simulink model "Simulink"  (R2023b)
settings: Solver=VariableStepAuto  StartTime=0.0  StopTime=1  RelTol=1e-3
undefined symbols (not defined in the file): gray, Rec, SDTV
libraries: visiongeotforms x6, visiontransforms x5, visionconversions x4, visionsources x2
settings Model: Creator=Omer  LastModifiedBy=Omer

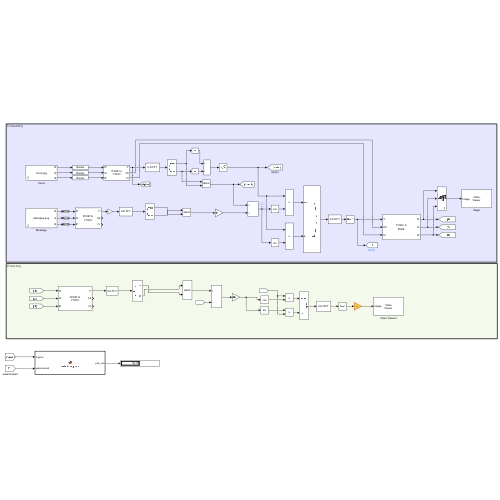
[thumbnail: Simulink's stored preview of the top-level diagram]
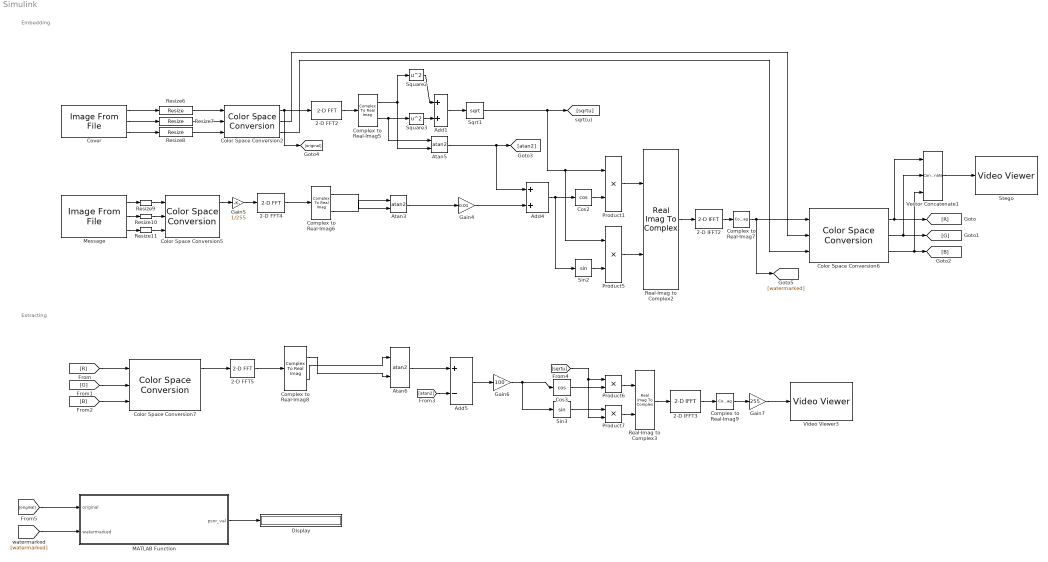
== system Simulink ==
  note: Extracting
  note: Embedding
  2-D FFT2 : visiontransforms/2-D FFT  TableOpt=NEW  TableOptActive=Speed  FFTImplementation=FFTW  BitRevOrder=off  SkipNorm=off  firstCoeffLastDataTypeStr=Inherit: Same word length as input  roundingMode=Floor  overflowMode=off  firstCoeffDataTypeStr=Inherit: Same word length as input  outputMin=[]  outputMax=[]
  2-D FFT4 : visiontransforms/2-D FFT  TableOpt=NEW  TableOptActive=Speed  FFTImplementation=FFTW  BitRevOrder=off  SkipNorm=off  firstCoeffLastDataTypeStr=Inherit: Same word length as input  roundingMode=Floor  overflowMode=off  firstCoeffDataTypeStr=Inherit: Same word length as input  outputMin=[]  outputMax=[]
  2-D FFT5 : visiontransforms/2-D FFT  TableOpt=NEW  TableOptActive=Speed  FFTImplementation=FFTW  BitRevOrder=off  SkipNorm=off  firstCoeffLastDataTypeStr=Inherit: Same word length as input  roundingMode=Floor  overflowMode=off  firstCoeffDataTypeStr=Inherit: Same word length as input  outputMin=[]  outputMax=[]
  2-D IFFT2 : visiontransforms/2-D IFFT  TableOpt=NEW  TableOptActive=Speed  FFTImplementation=FFTW  BitRevOrder=off  cs_in=off  divideOutput=on  SkipNorm=on  firstCoeffLastDataTypeStr=Inherit: Same word length as input  roundingMode=Floor  overflowMode=off  firstCoeffDataTypeStr=Inherit: Same word length as input  outputMin=[]  outputMax=[]
  2-D IFFT3 : visiontransforms/2-D IFFT  TableOpt=NEW  TableOptActive=Speed  FFTImplementation=FFTW  BitRevOrder=off  cs_in=off  divideOutput=on  SkipNorm=on  firstCoeffLastDataTypeStr=Inherit: Same word length as input  roundingMode=Floor  overflowMode=off  firstCoeffDataTypeStr=Inherit: Same word length as input  outputMin=[]  outputMax=[]
  Add1 : Sum
  Add4 : Sum
  Add5 : Sum  Inputs=+-
  Atan3 : Trigonometry  Operator=atan2
  Atan5 : Trigonometry  Operator=atan2
  Atan6 : Trigonometry  Operator=atan2
  Color Space Conversion2 : visionconversions/Color Space  Conversion  conversion=Obsolete  conversionActive=R'G'B' to Y'CbCr  wp_str=D65  rec=Rec. 601 (SDTV)  sys=1125/60/2:1  imagePorts=Separate color signals
  Color Space Conversion5 : visionconversions/Color Space  Conversion  conversion=Obsolete  conversionActive=R'G'B' to Y'CbCr  wp_str=D65  rec=Rec. 601 (SDTV)  sys=1125/60/2:1  imagePorts=Separate color signals
  Color Space Conversion6 : visionconversions/Color Space  Conversion  conversion=Obsolete  conversionActive=Y'CbCr to R'G'B'  wp_str=D65  rec=Rec. 601 (SDTV)  sys=1125/60/2:1  imagePorts=Separate color signals
  Color Space Conversion7 : visionconversions/Color Space  Conversion  conversion=Obsolete  conversionActive=R'G'B' to Y'CbCr  wp_str=D65  rec=Rec. 601 (SDTV)  sys=1125/60/2:1  imagePorts=Separate color signals
  Complex to Real-Imag5 : ComplexToRealImag
  Complex to Real-Imag6 : ComplexToRealImag
  Complex to Real-Imag7 : ComplexToRealImag  Output=Real
  Complex to Real-Imag8 : ComplexToRealImag
  Complex to Real-Imag9 : ComplexToRealImag  Output=Real
  Cos2 : Trigonometry  Operator=cos
  Cos3 : Trigonometry  Operator=cos
  Cover : visionsources/Image From File  Tag=vipblks_nd  FileName=C:\Users\Omer\Desktop\media\Cover.jpg  Ts=inf  imagePorts=Separate color signals  OutPortLabels=R|G|B  ImageDataType=double  sdImageDataType=uint(8)  Signed=on  WordLength=16  FractionLengthMode=User-defined  FractionLength=15
  Display : Display
  Gain4 : Gain  Gain=0.01
  Gain5 : Gain  Gain=1/255  ParamDataTypeStr=double  RndMeth=Nearest
  Gain6 : Gain  Gain=100
  Gain7 : Gain  Gain=255  OutDataTypeStr=uint8  SaturateOnIntegerOverflow=on
  MATLAB Function : MATLAB Function  TreatAsAtomicUnit=on
  Message : visionsources/Image From File  Tag=vipblks_nd  FileName=C:\Users\Omer\Desktop\media\Message.png  Ts=inf  imagePorts=Separate color signals  OutPortLabels=R|G|B  ImageDataType=double  sdImageDataType=uint(8)  Signed=on  WordLength=16  FractionLengthMode=User-defined  FractionLength=15
  Product{1,5..7} (4 alike) : Product
  Real-Imag to Complex2 : RealImagToComplex
  Real-Imag to Complex3 : RealImagToComplex
  Resize{6..11} (6 alike) : visiongeotforms/Resize  specify=Number of output rows and columns  rfactor=[512 512]  outCols=25  outRows=25  outRowsCols=[512 512]  interp_method=Bilinear  antialias=on  useROI=off  roiFlag=off  roundingMode=Nearest  overflowMode=on  prodOutputMode=Binary point scaling  prodOutputWordLength=32  prodOutputFracLength=10
  Sin2 : Trigonometry
  Sin3 : Trigonometry
  Sqrt1 : Sqrt
  Square2 : Math  Operator=square
  Square3 : Math  Operator=square
  Stego : VideoViewer  colormapValue=gray(256)  FigPos=[1 822 1536 724]
  Vector Concatenate1 : Concatenate  NumInputs=3  Mode=Multidimensional array  ConcatenateDimension=3
  Video Viewer3 : VideoViewer  colormapValue=gray(256)  FigPos=[1 822 1536 724]
  wires:
  Resize8/1 -> Color Space Conversion2/3
  Resize9/1 -> Color Space Conversion5/1
  Gain5/1 -> 2-D FFT4/1
  Message/1 -> Resize9/1
  Color Space Conversion2/2 -> Color Space Conversion6/2
  Cover/3 -> Resize8/1
  Atan3/1 -> Gain4/1
  Square2/1 -> Add1/1
  Square3/1 -> Add1/2
  Message/3 -> Resize11/1
  Resize7/1 -> Color Space Conversion2/2
  Complex to Real-Imag6/2 -> Atan3/1
  Add1/1 -> Sqrt1/1
  Product1/1 -> Real-Imag to Complex2/1
  Vector Concatenate1/1 -> Stego/1
  Sin2/1 -> Product5/2
  Resize11/1 -> Color Space Conversion5/3
  Complex to Real-Imag5/2 -> Atan5/1, Square3/1
  Message/2 -> Resize10/1
  Sqrt1/1 -> [sqrtu], Product1/1, Product5/1
  Cover/1 -> Resize6/1
  Product5/1 -> Real-Imag to Complex2/2
  Real-Imag to Complex2/1 -> 2-D IFFT2/1
  Atan5/1 -> [atan2], Add4/1
  Color Space Conversion5/1 -> Gain5/1
  Complex to Real-Imag5/1 -> Square2/1, Atan5/2
  2-D FFT2/1 -> Complex to Real-Imag5/1
  Cover/2 -> Resize7/1
  2-D FFT4/1 -> Complex to Real-Imag6/1
  2-D IFFT2/1 -> Complex to Real-Imag7/1
  Color Space Conversion2/3 -> Color Space Conversion6/3
  Add4/1 -> Cos2/1, Sin2/1
  Complex to Real-Imag7/1 -> [watermarked], Color Space Conversion6/1
  Complex to Real-Imag6/1 -> Atan3/2
  Cos2/1 -> Product1/2
  Color Space Conversion2/1 -> [original], 2-D FFT2/1
  Resize6/1 -> Color Space Conversion2/1
  Gain4/1 -> Add4/2
  Resize10/1 -> Color Space Conversion5/2
  Gain6/1 -> Sin3/1, Cos3/1
  Gain7/1 -> Video Viewer3/1
  Product7/1 -> Real-Imag to Complex3/2
  Complex to Real-Imag9/1 -> Gain7/1
  2-D FFT5/1 -> Complex to Real-Imag8/1
  [R] -> Color Space Conversion7/1
  Real-Imag to Complex3/1 -> 2-D IFFT3/1
  Product6/1 -> Real-Imag to Complex3/1
  Cos3/1 -> Product6/2
  2-D IFFT3/1 -> Complex to Real-Imag9/1
  Color Space Conversion7/1 -> 2-D FFT5/1
  Add5/1 -> Gain6/1
  Atan6/1 -> Add5/1
  [B] -> Color Space Conversion7/3
  Sin3/1 -> Product7/1
  Complex to Real-Imag8/2 -> Atan6/1
  [G] -> Color Space Conversion7/2
  Complex to Real-Imag8/1 -> Atan6/2
  Color Space Conversion6/1 -> Vector Concatenate1/1, [R]
  Color Space Conversion6/2 -> Vector Concatenate1/2, [G]
  Color Space Conversion6/3 -> Vector Concatenate1/3, [B]
  [atan2] -> Add5/2
  [sqrtu] -> Product7/2, Product6/1
  [original] -> MATLAB Function/1(original)
  [watermarked] -> MATLAB Function/2(watermarked)
  MATLAB Function/1(psnr_val) -> Display/1

== matlab function Simulink/MATLAB Function ==
  data: original input; psnr_val output; watermarked input
function psnr_val = calculate_psnr(original, watermarked)

    img1 = double(original);
    img2 = double(watermarked);
    

    [M, N] = size(img1);
    
    error = img1 - img2;
    mse = sum(sum(error .^ 2)) / (M * N);
    

    if mse == 0
        psnr_val = 100;
    else

        max_pixel = 1;
        psnr_val = 10 * log10((max_pixel^2) / mse);
    end
end
